simulink model "Real_proc_LinuxMPC"  (Simulink 7.9)
settings: Solver=ode45  StartTime=0.0  StopTime=60  RelTol=1e-3
values from neighbouring files (symbols this model uses):
  h = Ts_kalman    (= 0.01)    [MPC_setup_nonlinear.m]    (also in real_phi_ref.mat; real_phi_ref_2.mat; real_phi_ref_temp.mat; real_theta_constraint.mat)
  P_0 = eye(8)*100    [MPC_setup_nonlinear.m]    (also in real_phi_ref.mat = [100 0 0 0 0 0 0 0 0 100 0 0 ... (64 elements, 8x8)]; real_phi_ref_2.mat = [100 0 0 0 0 0 0 0 0 100 0 0 ... (64 elements, 8x8)]; real_phi_ref_temp.mat = [100 0 0 0 0 0 0 0 0 100 0 0 ... (64 elements, 8x8)]; real_theta_constraint.mat = [100 0 0 0 0 0 0 0 0 100 0 0 ... (64 elements, 8x8)])
  R1 = sqrtm(R)    [MPC_setup_nonlinear.m]    (also in real_phi_ref.mat = [0.00081901538426  9.06300190075e-05; 9.06300190075e-05  0.0; real_phi_ref_2.mat = [0.00081901538426  9.06300190075e-05; 9.06300190075e-05  0.0; real_phi_ref_temp.mat = [0.00081901538426  9.06300190075e-05; 9.06300190075e-05  0.0; real_theta_constraint.mat = [0.00081901538426  9.06300190075e-05; 9.06300190075e-05  0.0)
  Ts_control = 0.02    [MPC_setup_nonlinear.m]    (also in real_phi_ref.mat; real_phi_ref_2.mat; real_phi_ref_temp.mat; real_theta_constraint.mat)
  Ts_kalman = 0.01    [MPC_setup_nonlinear.m]    (also in real_phi_ref.mat; real_phi_ref_2.mat; real_phi_ref_temp.mat; real_theta_constraint.mat)
  x_0 = [0,-pi/4,0,0,0,0,0,0]    [MPC_setup_nonlinear.m]    (also in real_phi_ref.mat = [0 -0.785398163397 0 0 0 0 0 0]; real_phi_ref_2.mat = [0 -0.785398163397 0 0 0 0 0 0]; real_phi_ref_temp.mat = [0 -0.785398163397 0 0 0 0 0 0]; real_theta_constraint.mat = [0 -0.785398163397 0 0 0 0 0 0])
libraries: simulink x3
settings Model: Creator=tna13skn  LastModifiedBy=dat14rsa

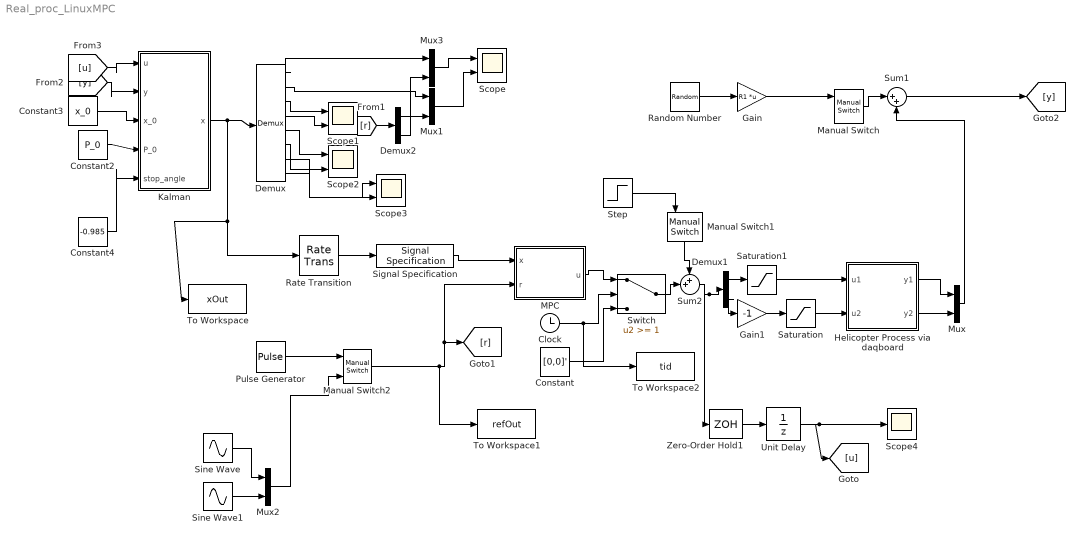
== system Real_proc_LinuxMPC ==
  Clock : Clock
  Constant : Constant  Value=[0,0]'
  Constant2 : Constant  Value=P_0  VectorParams1D=off  SampleTime=Ts_kalman
  Constant3 : Constant  Value=x_0  SampleTime=Ts_kalman
  Constant4 : Constant  Value=-0.985  SampleTime=Ts_kalman
  Demux : Demux  Outputs=8
  Demux1 : Demux  Outputs=2
  Demux2 : Demux  Outputs=2
  Gain : Gain  Gain=R1  Multiplication=Matrix(K*u)
  Gain1 : Gain  Gain=-1
  Helicopter Process via daqboard : Subsystem
  Kalman : MATLAB Function  TreatAsAtomicUnit=on
  MPC : MATLAB Function  TreatAsAtomicUnit=on
  Manual Switch : simulink/Signal Routing/Manual Switch  sw=0  action=0  varsize=off
  Manual Switch1 : simulink/Signal Routing/Manual Switch  sw=0  action=0  varsize=off
  Manual Switch2 : simulink/Signal Routing/Manual Switch  sw=1  action=0  varsize=off
  Mux{,1..3} (4 alike) : Mux  Inputs=2
  Pulse Generator : DiscretePulseGenerator  Amplitude=[-0.7 0]'  Period=30/Ts_control  PulseWidth=15/Ts_control  SampleTime=Ts_control
  Random Number : RandomNumber  Mean=[0,0]'  Variance=[1,1]'  Seed=[1,3]  SampleTime=Ts_kalman
  Rate Transition : RateTransition  X0=x_0  OutPortSampleTime=Ts_control
  Saturation : Saturate  UpperLimit=10  LowerLimit=-10
  Saturation1 : Saturate  UpperLimit=10  LowerLimit=-10
  Scope{,1..3} (4 alike) : Scope  NumInputPorts=2
      Scope settings: TimeRange=60  YMin=-1.2~-1  YMax=0.1~0.1
      Scope1 settings: YMin=-5~-5  YMax=5~5
      Scope2 settings: YMin=-5~-5  YMax=5~5  SaveName=ScopeData2
      Scope3 settings: YMin=-0.4~-2  YMax=0.35~1  SaveName=ScopeData3
  Scope4 : Scope
      settings: YMin=-4  YMax=3  SaveName=ScopeData4
  Signal Specification : SignalSpecification  Dimensions=[8,1]  SampleTime=Ts_control
      settings: LockScale=on
  Sine Wave : Sin  Amplitude=1.5  Frequency=0.5  SampleTime=Ts_control
  Sine Wave1 : Sin  Amplitude=0.4  Frequency=0.5  SampleTime=Ts_control
  Step : Step  Time=30  Before=[0,0]'  After=[1,1]'*0.3  SampleTime=0
  Sum1 : Sum  Inputs=|++
  Sum2 : Sum  Inputs=++|
  Switch : Switch  Threshold=1
  To Workspace : ToWorkspace  VariableName=xOut  SampleTime=-1  SaveFormat=Timeseries
  To Workspace1 : ToWorkspace  VariableName=refOut  SampleTime=-1  SaveFormat=Timeseries
  To Workspace2 : ToWorkspace  VariableName=tid  SampleTime=-1  SaveFormat=Timeseries
  Unit Delay : UnitDelay  SampleTime=-1
  Zero-Order Hold1 : ZeroOrderHold  SampleTime=Ts_kalman
  wires:
  Kalman/1(x) -> Demux/1, Rate Transition/1, To Workspace/1
  Demux/3 -> Scope1/1
  Demux/4 -> Scope1/2
  Demux/5 -> Scope2/1
  Demux/6 -> Scope2/2
  Rate Transition/1 -> Signal Specification/1
  Signal Specification/1 -> MPC/1(x)
  MPC/1(u) -> Switch/1
  Clock/1 -> Switch/2, To Workspace2/1
  Constant/1 -> Switch/3
  Demux/7 -> Scope3/1
  Demux/8 -> Scope3/2
  Zero-Order Hold1/1 -> Unit Delay/1
  Unit Delay/1 -> Scope4/1, [u]
  Random Number/1 -> Gain/1
  Gain/1 -> Manual Switch/1
  Sum1/1 -> [y]
  Sum2/1 -> Zero-Order Hold1/1, Demux1/1
  Manual Switch1/1 -> Sum2/1
  Step/1 -> Manual Switch1/1
  Manual Switch2/1 -> [r], MPC/2(r), To Workspace1/1
  Pulse Generator/1 -> Manual Switch2/1
  Constant2/1 -> Kalman/4(P_0)
  Constant3/1 -> Kalman/3(x_0)
  [y] -> Kalman/2(y)
  [u] -> Kalman/1(u)
  Constant4/1 -> Kalman/5(stop_angle)
  Switch/1 -> Sum2/2
  Manual Switch/1 -> Sum1/1
  Demux1/1 -> Saturation1/1
  Helicopter Process via daqboard/1(y1) -> Mux/1
  Helicopter Process via daqboard/2(y2) -> Mux/2
  Mux/1 -> Sum1/2
  Saturation1/1 -> Helicopter Process via daqboard/1(u1)
  Saturation/1 -> Helicopter Process via daqboard/2(u2)
  Demux/2 -> Mux1/1
  [r] -> Demux2/1
  Demux2/2 -> Mux1/2
  Mux1/1 -> Scope/2
  Sine Wave1/1 -> Mux2/2
  Sine Wave/1 -> Mux2/1
  Mux2/1 -> Manual Switch2/2
  Gain1/1 -> Saturation/1
  Demux1/2 -> Gain1/1
  Demux/1 -> Mux3/1
  Demux2/1 -> Mux3/2
  Mux3/1 -> Scope/1

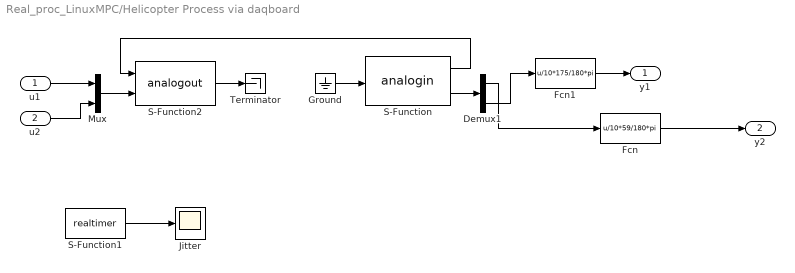
== system Real_proc_LinuxMPC/Helicopter Process via daqboard ==
  u1 : Inport
  u2 : Inport  Port=2
  Demux1 : Demux  Outputs=2
  Fcn : Fcn  Expr=u/10*59/180*pi
  Fcn1 : Fcn  Expr=u/10*175/180*pi
  Ground : Ground
  Jitter : Scope
  Mux : Mux  Inputs=2
  S-Function : S-Function  FunctionName=analogin  Parameters=h [0 1]  EnableBusSupport=off
  S-Function1 : S-Function  FunctionName=realtimer  Parameters=h  EnableBusSupport=off
  S-Function2 : S-Function  FunctionName=analogout  Parameters=h [0 1]  EnableBusSupport=off
  Terminator : Terminator
  y1 : Outport  InitialOutput=0
  y2 : Outport  Port=2  InitialOutput=0
  wires:
  S-Function1/1 -> Jitter/1
  Mux/1 -> S-Function2/2
  Demux1/2 -> Fcn1/1
  Demux1/1 -> Fcn/1
  S-Function/2 -> Demux1/1
  u2/1 -> Mux/2
  u1/1 -> Mux/1
  Ground/1 -> S-Function/1
  S-Function2/1 -> Terminator/1
  S-Function/1 -> S-Function2/1
  Fcn/1 -> y2/1
  Fcn1/1 -> y1/1

== matlab function MPC ==
  data: u output double; x input double; r input double
function u = MPC(x,r)
coder.extrinsic('mycsolve');
u=[0;0];
u=mycsolve(x,r);
end

== matlab function Kalman ==
  data: u input double; y input double; x_0 input double; P_0 input double; stop_angle input double; x output double
function x = kalman(u,y,x_0,P_0,stop_angle)

persistent x_hat;
persistent P;
if(isempty(x_hat))
    x_hat=x_0;
    P=P_0;
end
coder.extrinsic('updateKalman');

[x_hat,P]=updateKalman(x_hat,u,y,P,stop_angle);

x=x_hat;
